simulink model "Full_Bridge_Inverter_Correct"  (R2021b)
settings: Solver=VariableStepAuto  StartTime=0.0  StopTime=1  RelTol=1e-3
libraries: spsMosfetLib x4, spsSeriesRLCBranchLib x3, spsVoltageMeasurementLib x2, spsDCVoltageSourceLib x1, spsRMSLib x1, spsTriangleGeneratorLib x1, spspowerguiLib x1
settings Model: Creator=nandi  LastModifiedBy=nandi
settings DataIOCC: ReturnWorkspaceOutputs=off

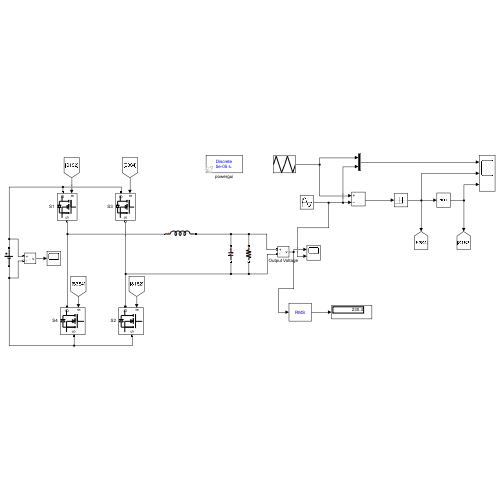
[thumbnail: Simulink's stored preview of the top-level diagram]
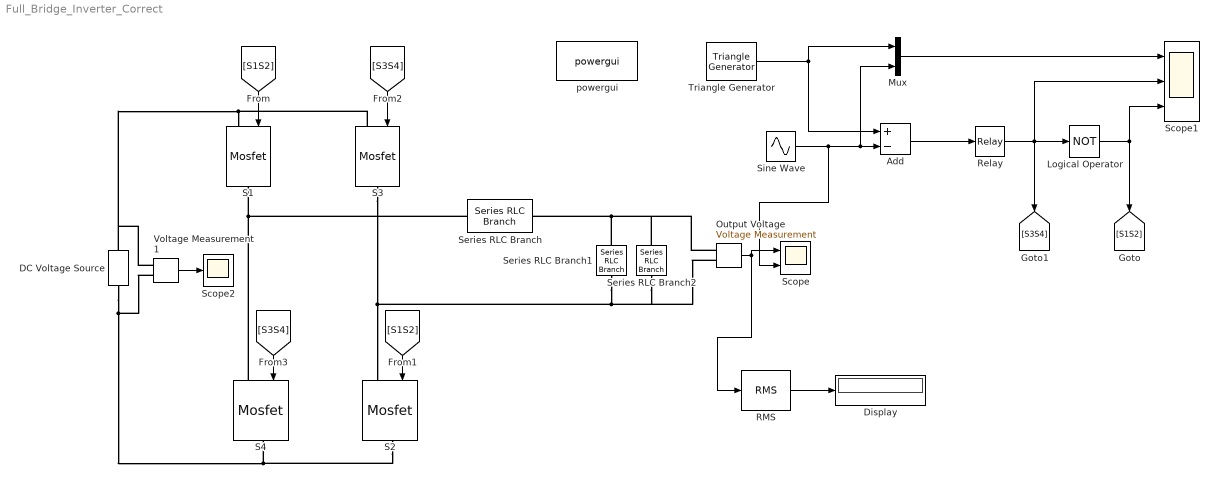
== system Full_Bridge_Inverter_Correct ==
  Add : Sum  Inputs=+-
  DC Voltage Source : spsDCVoltageSourceLib/DC Voltage Source  Amplitude=400  Measurements=None
  Display : Display
  Logical Operator : Logic  Operator=NOT  AllPortsSameDT=off  OutDataTypeStr=boolean
  Mux : Mux  Inputs=2
  Output Voltage : spsVoltageMeasurementLib/Voltage Measurement  PhasorSimulation=off  OutputType=Complex  PSBequivalent=0
  RMS : spsRMSLib/RMS  TrueRMS=on  Freq=50  RMSInit=120  Ts=0
  Relay : Relay
  S{1..4} (4 alike) : spsMosfetLib/Mosfet  Ron=0.1  Lon=0  Rd=0.01  Vfd=0  IC=0  Rs=1e5  Cs=inf  Measurements=off
  Scope : Scope  NumInputPorts=2
  Scope1 : Scope  NumInputPorts=3
  Scope2 : Scope
  Series RLC Branch : spsSeriesRLCBranchLib/Series RLC Branch  LConnTagsString=__new0  RConnTagsString=__new0  BranchType=L  Resistance=1  Inductance=1e-3  SetiL0=off  InitialCurrent=0  Capacitance=1e-6  Setx0=off  InitialVoltage=0  Measurements=None
  Series RLC Branch1 : spsSeriesRLCBranchLib/Series RLC Branch  LConnTagsString=__new0  RConnTagsString=__new0  BranchType=C  Resistance=1  Inductance=1e-3  SetiL0=off  InitialCurrent=0  Capacitance=6e-3  Setx0=off  InitialVoltage=0  Measurements=None
  Series RLC Branch2 : spsSeriesRLCBranchLib/Series RLC Branch  LConnTagsString=__new0  RConnTagsString=__new0  BranchType=R  Resistance=0.364  Inductance=1e-3  SetiL0=off  InitialCurrent=0  Capacitance=6e-3  Setx0=off  InitialVoltage=0  Measurements=None
  Sine Wave : Sin  Frequency=2*pi*50  SampleTime=0
  Triangle Generator : spsTriangleGeneratorLib/Triangle Generator  Freq=100e3  Phase=90  Ts=0
  Voltage Measurement1 : spsVoltageMeasurementLib/Voltage Measurement  PhasorSimulation=off  OutputType=Complex  PSBequivalent=0
  powergui : spspowerguiLib/powergui  Priority=1  SimulationMode=Discrete  SampleTime=50e-6  frequency=60  Iterations=50  frequencyindice=0  Pbase=100e6  ErrMax=1e-4  UnitsV=kV  UnitsW=MW  buscounter=0  FunctionMessages=off  echomessages=off  EnableUseOfTLC=off  CurrentSourceSwitches=off  DisableSnubberDevices=off  DisableRonSwitches=off  DisableVfSwitches=off  DisplayEquations=off  AutomaticDiscreteSolvers=off  SolverType=Tustin/Backward Euler (TBE)  Interpol=off  ExternalGateDelay=off  methode=off  Ts=100  x0status=blocks  SPID=on  SwTol=0  HookPort=off  NonlinearTolerance=1e-4  nMaxIteration=100  ContinueOnMaxIteration=off  RestoreLinks=warning  ResistiveCurrentMeasurement=off  Frange=[0:2:500]  Ylog=off  Xlog=on  ShowGrid=off  save=off  variable=ZData  structure=0  ZoomFFT=off  StartTime=0.0  cycles=1  DisplayStyle=1  fundamental=60  FreqAxis=off  MaxFrequency=1000  frequencyindicesteady=1  RmsSteady=1  display=off
  wires:
  Output Voltage/1 -> RMS/1, Scope/1
  Sine Wave/1 -> Scope/2, Mux/2, Add/2
  Add/1 -> Relay/1
  Relay/1 -> Logical Operator/1, [S3S4], Scope1/2
  Logical Operator/1 -> [S1S2], Scope1/3
  Mux/1 -> Scope1/1
  [S1S2] -> S1/1
  [S1S2] -> S2/1
  [S3S4] -> S3/1
  [S3S4] -> S4/1
  Voltage Measurement1/1 -> Scope2/1
  RMS/1 -> Display/1
  Triangle Generator/1 -> Add/1, Mux/1
  connections:
  S3/LConn1 -- Voltage Measurement1/LConn1 -- DC Voltage Source/RConn1 -- S1/LConn1
  DC Voltage Source/LConn1 -- Voltage Measurement1/LConn2 -- S2/RConn1 -- S4/RConn1
  S4/LConn1 -- Series RLC Branch/LConn1 -- S1/RConn1
  S3/RConn1 -- Series RLC Branch2/RConn1 -- Output Voltage/LConn2 -- Series RLC Branch1/RConn1 -- S2/LConn1
  Series RLC Branch1/LConn1 -- Series RLC Branch2/LConn1 -- Output Voltage/LConn1 -- Series RLC Branch/RConn1
